simulink model "cube3d_simulation_linearized"  (R2016a)
settings: Solver=VariableStepAuto  StartTime=0.0  StopTime=10.0  RelTol=1e-3
values from neighbouring files (symbols this model uses):
  K_lqr_3D = [0.287489072363 0.287489072363 0.238143218168 4.56359884784 -4.56359884784 3.24507356919e-15 -1.59498144248 -1.59498144248 4.58035976599 0.296440037514 0.296440037514 0.246356019125 ... (18 elements, 3x6)]    [K_lqr_3D.mat]
  sys_d = c2d(sys_c, Ts)    [LQR_2d.m]    (also in LQR_3d.m)
  Ts = 0.001    [LQR_2d.m]    (also in LQR_3d.m = 0.002; Linearized_system.m; cubeparameters.m = struct('controller',  0.024,              'IMU',         0.0)
  x0 = [pi/4 ; 0 ]    [LQR_2d.m]    (also in LQR_3d.m = [0.1,0.1,0.1,0,0,5]; run_simulation_2D.m = [deg2rad(2) ; 0]; testa.m = zeros(3,1))
settings Model: Creator=Love  LastModifiedBy=Love

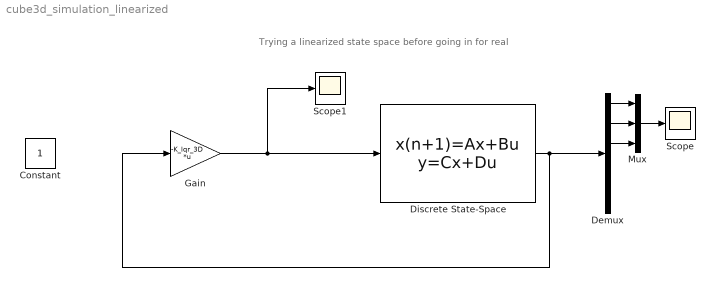
== system cube3d_simulation_linearized ==
  note: Trying a linearized state space before going in for real
  Constant : Constant
  Demux : Demux  Outputs=6
  Discrete State-Space : DiscreteStateSpace  A=sys_d.A  B=sys_d.B  C=sys_d.C  D=zeros(6,3)  X0=x0  SampleTime=Ts
  Gain : Gain  Gain=-K_lqr_3D  Multiplication=Matrix(K*u)
  Mux : Mux  Inputs=3
  Scope : Scope
  Scope1 : Scope
  wires:
  Gain/1 -> Scope1/1, Discrete State-Space/1
  Discrete State-Space/1 -> Demux/1, Gain/1
  Demux/1 -> Mux/1
  Demux/2 -> Mux/2
  Demux/3 -> Mux/3
  Mux/1 -> Scope/1
